simulink model "LUGOT"  (R2021a)
settings: Solver=FixedStepDiscrete  StartTime=0.0  StopTime=length(time_uwb)-1  FixedStep=Ts  MaxStep=Ts  RelTol=1e-3
values from neighbouring files (symbols this model uses):
  a = (vx .* ax + vy .* ay) ./ v    [relative_spd_vs_residual.m]    (also in smoothing_spline_fit.m)
  num_init_steps = uint8(3)    [main.m]
  outlier_threshold = standerd_deviation * 3.75 * 2 + 0.0    [main.m]
  Ts = 1.    (= 1)    [main.m]    (also in stateTransitionFcn_PF.m = 0.01)
undefined symbols (not defined in the file or in its folder): delta_h, Discrete, Time
libraries: sharedTrackingLibrary x9, simulink x6, dspstat3 x4, ctrlSharedLib x1
(part 2 of 2)

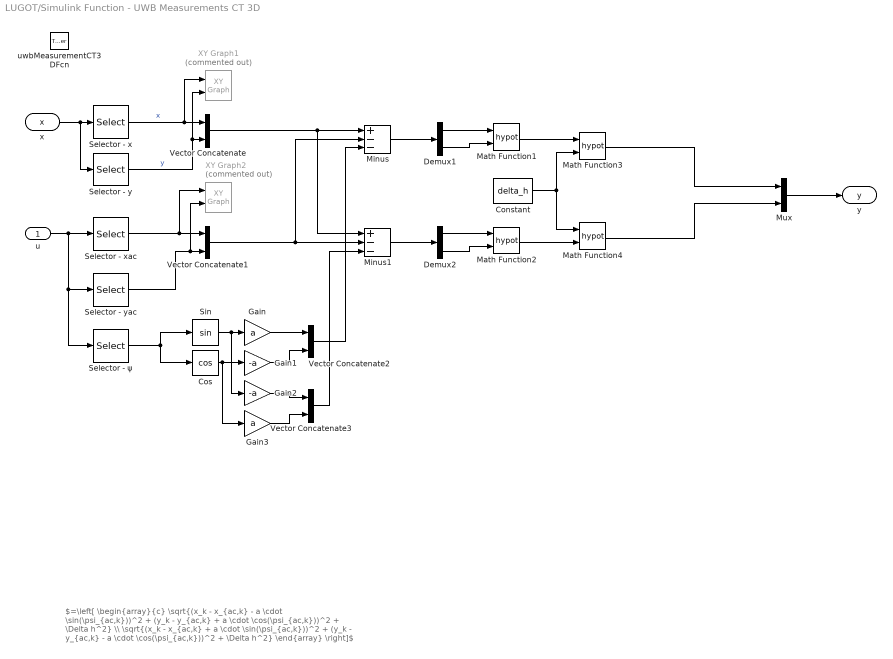
== system LUGOT/Simulink Function - UWB Measurements CT 3D ==
  note: $=\left[ \begin{array}{c} \sqrt{(x_k - x_{ac,k} - a \cdot \sin(\psi_{ac,k}))^2 + (y_k - y_{ac,k} + a \cdot \cos(\psi_{ac,k}))^2 + \Delta h^2} \\ \sqrt{(x_k - x_{ac,k} + a \cdot \sin(\psi_{ac,k}))^2 + (y_k - y_{ac,k} - a \cdot \cos(\psi_{ac,k}))^2 + \Delta h^2} \end{array} \right]$
  u : Inport
  uwbMeasurementCT3DFcn : TriggerPort  TriggerType=function-call  IsSimulinkFunction=on  FunctionName=uwbMeasurementCT3DFcn  VariantControl=Variant
  Constant : Constant  Value=delta_h
  Cos : Trigonometry  Operator=cos
  Demux1 : Demux  Outputs=2
  Demux2 : Demux  Outputs=2
  Gain : Gain  Gain=a
  Gain1 : Gain  Gain=-a
  Gain2 : Gain  Gain=-a
  Gain3 : Gain  Gain=a
  Math Function{1..4} (4 alike) : Math  Operator=hypot  SignedPower=on  SaturateOnIntegerOverflow=on
  Minus : Sum  Inputs=+--
  Minus1 : Sum  Inputs=+--
  Mux : Mux  Inputs=2
  Selector - x : Selector  InputPortWidth=5  IndexOptions=Index vector (dialog)  Indices=1  OutputSizes=1
  Selector - xac : Selector  InputPortWidth=3  IndexOptions=Index vector (dialog)  Indices=1  OutputSizes=1
  Selector - y : Selector  InputPortWidth=5  IndexOptions=Index vector (dialog)  Indices=3  OutputSizes=1
  Selector - yac : Selector  InputPortWidth=3  IndexOptions=Index vector (dialog)  Indices=2  OutputSizes=1
  Selector - ψ : Selector  InputPortWidth=3  IndexOptions=Index vector (dialog)  Indices=3  OutputSizes=1
  Sin : Trigonometry
  Vector Concatenate{,1..3} (4 alike) : Concatenate
  XY Graph1 : simulink/Sinks/XY Graph  Commented=on  xmin=0  xmax=220  ymin=-17  ymax=34  st=-1
  XY Graph2 : simulink/Sinks/XY Graph  Commented=on  xmin=0  xmax=220  ymin=-17  ymax=34  st=-1
  x : ArgIn  DisableCoverage=on  PortDimensions=5  ArgumentName=x
  y : ArgOut  DisableCoverage=on  PortDimensions=2  ArgumentName=y
  wires:
  Mux/1 -> y/1
  Minus1/1 -> Demux2/1
  Demux2/1 -> Math Function2/1
  Demux2/2 -> Math Function2/2
  Demux1/2 -> Math Function1/2
  Demux1/1 -> Math Function1/1
  Minus/1 -> Demux1/1
  Vector Concatenate3/1 -> Minus1/3
  Vector Concatenate2/1 -> Minus/3
  Vector Concatenate1/1 -> Minus1/2, Minus/2
  Vector Concatenate/1 -> Minus/1, Minus1/1
  Gain2/1 -> Vector Concatenate3/1
  Cos/1 -> Gain1/1, Gain3/1
  Sin/1 -> Gain/1, Gain2/1
  Gain3/1 -> Vector Concatenate3/2
  Gain1/1 -> Vector Concatenate2/2
  Gain/1 -> Vector Concatenate2/1
  Selector - ψ/1 -> Cos/1, Sin/1
  Selector - yac/1 -> Vector Concatenate1/2, XY Graph2/2
  Selector - xac/1 -> Vector Concatenate1/1, XY Graph2/1
  u/1 -> Selector - xac/1, Selector - yac/1, Selector - ψ/1
  x/1 -> Selector - x/1, Selector - y/1
  Selector - y/1 -> Vector Concatenate/2, XY Graph1/2  "y"
  Selector - x/1 -> Vector Concatenate/1, XY Graph1/1  "x"
  Math Function1/1 -> Math Function3/1
  Math Function2/1 -> Math Function4/2
  Constant/1 -> Math Function3/2, Math Function4/1
  Math Function3/1 -> Mux/1
  Math Function4/1 -> Mux/2

== system LUGOT/Subsystem ==
  Ts : Inport
  Constant1 : Constant  Value=[1 0 0 0; 0 1 0 0]  VectorParams1D=off
  MATLAB Function : MATLAB Function  TreatAsAtomicUnit=on
  MATLAB Function1 : MATLAB Function  TreatAsAtomicUnit=on
  A : Outport
  C : Outport  Port=2
  G : Outport  Port=3
  wires:
  MATLAB Function1/1(G) -> G/1
  Ts/1 -> MATLAB Function1/1(Ts), MATLAB Function/1(Ts)
  MATLAB Function/1(A) -> A/1
  Constant1/1 -> C/1

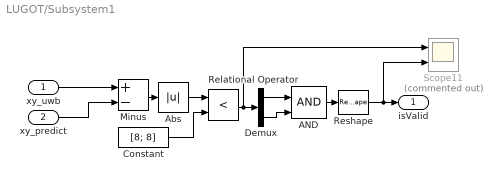
== system LUGOT/Subsystem1 ==
  xy_uwb : Inport
  xy_predict : Inport  Port=2
  AND : Logic  IconShape=distinctive  AllPortsSameDT=off  OutDataTypeStr=boolean
  Abs : Abs
  Constant : Constant  Value=[8; 8]
  Demux : Demux  Outputs=2
  Minus : Sum  Inputs=+-
  Relational Operator : RelationalOperator  Operator=<  OutDataTypeStr=boolean  RndMeth=Simplest
  Reshape : Reshape
  Scope11 : Scope  Commented=on  NumInputPorts=2
  isValid : Outport
  wires:
  Abs/1 -> Relational Operator/1
  AND/1 -> Reshape/1
  Demux/2 -> AND/2
  Constant/1 -> Relational Operator/2
  Relational Operator/1 -> Scope11/1, Demux/1
  Demux/1 -> AND/1
  xy_uwb/1 -> Minus/1
  Minus/1 -> Abs/1
  xy_predict/1 -> Minus/2
  Reshape/1 -> Scope11/2, isValid/1

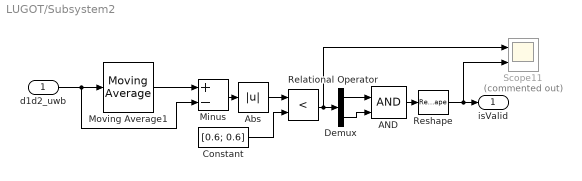
== system LUGOT/Subsystem2 ==
  d1d2_uwb : Inport
  AND : Logic  IconShape=distinctive  AllPortsSameDT=off  OutDataTypeStr=boolean
  Abs : Abs
  Constant : Constant  Value=[0.6; 0.6]
  Demux : Demux  Outputs=2
  Minus : Sum  Inputs=+-
  Moving Average1 : dspstat3/Moving Average  Method=Sliding window  ForgettingFactorPort=off  SpecifyWindowLength=on  WindowLength=20  ForgettingFactor=0.9  SimulateUsing=Code generation
  Relational Operator : RelationalOperator  Operator=<  OutDataTypeStr=boolean  RndMeth=Simplest
  Reshape : Reshape
  Scope11 : Scope  Commented=on  NumInputPorts=2
  isValid : Outport
  wires:
  Reshape/1 -> isValid/1, Scope11/2
  Minus/1 -> Abs/1
  Moving Average1/1 -> Minus/1
  Demux/1 -> AND/1
  Relational Operator/1 -> Demux/1, Scope11/1
  Constant/1 -> Relational Operator/2
  Demux/2 -> AND/2
  AND/1 -> Reshape/1
  Abs/1 -> Relational Operator/1
  d1d2_uwb/1 -> Minus/2, Moving Average1/1

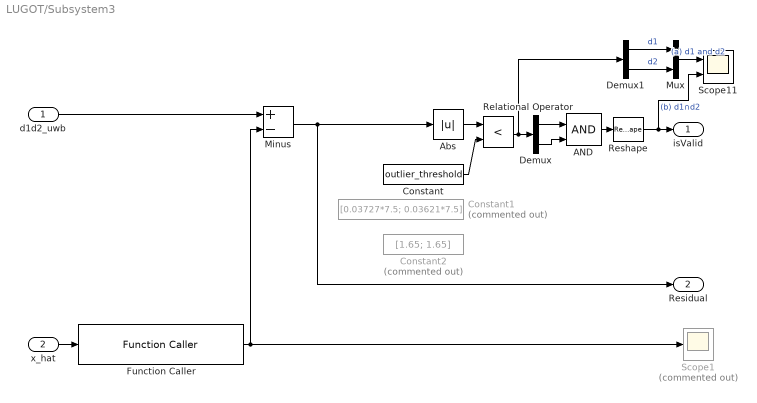
== system LUGOT/Subsystem3 ==
  d1d2_uwb : Inport
  x_hat : Inport  Port=2
  AND : Logic  IconShape=distinctive  AllPortsSameDT=off  OutDataTypeStr=boolean
  Abs : Abs
  Constant : Constant  Value=outlier_threshold
  Constant1 : Constant  Commented=on  Value=[0.03727*7.5; 0.03621*7.5]
  Constant2 : Constant  Commented=on  Value=[1.65; 1.65]
  Demux : Demux  Outputs=2
  Demux1 : Demux  Outputs=2
  Function Caller : FunctionCaller  FunctionPrototype=y = uwbMeasurementCT3DFcn(x)  InputArgumentSpecifications=<Enter example>  OutputArgumentSpecifications=<Enter example>
  Minus : Sum  Inputs=+-
  Mux : Mux  Inputs=2
  Relational Operator : RelationalOperator  Operator=<  OutDataTypeStr=boolean  RndMeth=Simplest
  Reshape : Reshape
  Scope1 : Scope  Commented=on
  Scope11 : Scope  NumInputPorts=2
  isValid : Outport
  Residual : Outport  Port=2
  wires:
  Abs/1 -> Relational Operator/1
  AND/1 -> Reshape/1
  Demux/2 -> AND/2
  Constant/1 -> Relational Operator/2
  Relational Operator/1 -> Demux1/1, Demux/1
  Demux/1 -> AND/1
  d1d2_uwb/1 -> Minus/1
  Minus/1 -> Abs/1, Residual/1
  Reshape/1 -> Scope11/2, isValid/1  "(b) d1∩d2"
  Function Caller/1 -> Scope1/1, Minus/2
  x_hat/1 -> Function Caller/1
  Mux/1 -> Scope11/1  "(a) d1 and d2"
  Demux1/1 -> Mux/1  "d1"
  Demux1/2 -> Mux/2  "d2"

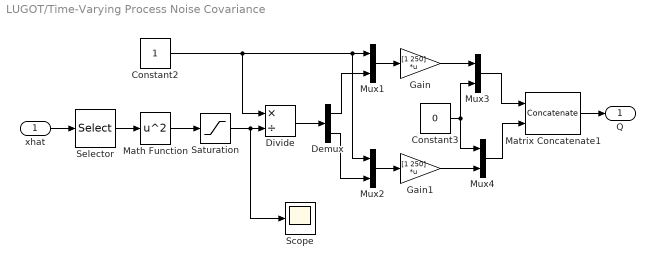
== system LUGOT/Time-Varying Process Noise Covariance ==
  xhat : Inport
  Constant2 : Constant
  Constant3 : Constant  Value=0
  Demux : Demux  Outputs=2
  Divide : Product  Inputs=*/
  Gain : Gain  Gain=[1 250]  Multiplication=Matrix(K*u)
  Gain1 : Gain  Gain=[1 250]  Multiplication=Matrix(K*u)
  Math Function : Math  Operator=square  SignedPower=on  SaturateOnIntegerOverflow=on
  Matrix Concatenate1 : Concatenate  Mode=Multidimensional array  ConcatenateDimension=2
  Mux{1..4} (4 alike) : Mux  Inputs=2
  Saturation : Saturate  UpperLimit=625  LowerLimit=25
  Scope : Scope
  Selector : Selector  InputPortWidth=4  IndexOptions=Index vector (dialog)  Indices=[3 4]  OutputSizes=1
  Q : Outport
  wires:
  Selector/1 -> Math Function/1
  xhat/1 -> Selector/1
  Saturation/1 -> Scope/1, Divide/2
  Constant2/1 -> Mux2/1, Mux1/1, Divide/1
  Divide/1 -> Demux/1
  Gain/1 -> Mux3/1
  Constant3/1 -> Mux3/2, Mux4/1
  Mux3/1 -> Matrix Concatenate1/1
  Mux4/1 -> Matrix Concatenate1/2
  Matrix Concatenate1/1 -> Q/1
  Demux/1 -> Mux1/2
  Demux/2 -> Mux2/2
  Mux1/1 -> Gain/1
  Mux2/1 -> Gain1/1
  Gain1/1 -> Mux4/2
  Math Function/1 -> Saturation/1

== system LUGOT/calc ΔT ==
  Time : Inport
  Enable : EnablePort
  Constant1 : Constant  Commented=on  Value=1/120
  Memory : Memory  InitialCondition=-1/120  InheritSampleTime=on
  Subtract : Sum  Inputs=+-
  Switch : Switch  Commented=on  Criteria=u2 > Threshold  Threshold=1e-3
  dt : Outport
  wires:
  Subtract/1 -> dt/1
  Time/1 -> Memory/1, Subtract/1
  Memory/1 -> Subtract/2
  ? -> Switch/1, Switch/2
  Constant1/1 -> Switch/3

== system LUGOT/calc ΔT1 ==
  Time : Inport
  Enable : EnablePort
  Memory : Memory  InitialCondition=-1/120  InheritSampleTime=on
  Subtract : Sum  Inputs=+-
  dt : Outport
  wires:
  Subtract/1 -> dt/1
  Time/1 -> Memory/1, Subtract/1
  Memory/1 -> Subtract/2

== system LUGOT/initial_counter ==
  Enable : EnablePort
  Add : Sum
  Constant : Constant
  Constant2 : Constant  Value=num_init_steps
  Memory2 : Memory  InheritSampleTime=on
  Relational Operator : RelationalOperator  Operator=>  OutDataTypeStr=boolean  RndMeth=Simplest
  Scope27 : Scope  Commented=on
  Out1 : Outport
  wires:
  Constant2/1 -> Relational Operator/2
  Constant/1 -> Add/1
  Add/1 -> Memory2/1, Scope27/1, Relational Operator/1
  Memory2/1 -> Add/2
  Relational Operator/1 -> Out1/1

== matlab function LUGOT/Simulink Function - State Transition CTRV/MATLAB Function ==
  data: current_state input; next_state output; dt input
% https://blog.csdn.net/west_gege/article/details/121405259
% function state  = predict_omega(state,dt)
%   % state = x,y,v,theta,omega
%   state(1) = state(1) + (state(3) / state(5)) * (sin(state(4) + state(5) * dt) - sin(state(4)));
%   state(2) = state(2) + (state(3) / state(5)) *(-cos(state(4) + state(5) * dt) + cos(state(4)));
%   state(3) = state(3);
%   state(4) = state(4) + state(5) * dt;
%   state(5) = state(5);
% end
% 
% function [state] = predict_omega(state,dt)
%     % state = x,y,v,theta,omega
%   state(1) = state(1) + state(3)*cos(state(4))*dt;
%   state(2) = state(2) + state(3)*sin(state(4))*dt;
%   state(3) = state(3);
%   state(4) = state(4);
%   state(5) = state(5);
% end

function next_state = ctrv_transition(current_state, dt)
    % 解析当前状态
    x = current_state(1);
    y = current_state(2);
    theta = current_state(3);
    v = current_state(4);
    omega = current_state(5);

    % 如果转向率非零，则使用CTRV模型进行状态更新
    if omega ~= 0
        % 计算新的位置和航向
        next_x = x + (v/omega) * (sin(theta + omega*dt) - sin(theta));
        next_y = y + (v/omega) * (cos(theta) - cos(theta + omega*dt));
        next_theta = theta + omega*dt;
    else
        % 当转向率为零时，退化为直线运动
        next_x = x + v*cos(theta)*dt;
        next_y = y + v*sin(theta)*dt;
        next_theta = theta;
    end

    % 更新速度和转向率（这里假设它们在时间间隔内保持不变）
    next_v = v;
    next_omega = omega;

    % 组合成新的状态向量
    next_state = [next_x; next_y; next_theta; next_v; next_omega];
end

== matlab function LUGOT/Simulink Function - State Transition CT/MATLAB Function ==
  data: x input; y output; w input; dt input
function y = stateTransitionCTFcn(x,w,dt)

y = constturn(x,w,dt); %0.01

== matlab function LUGOT/Simulink Function - State Transition Jacobian CT/MATLAB Function ==
  data: x input; A output; w input; G output; dt input
function [A,G] = fcn(x,w,dt)
[A,G] = constturnjac(x,w,dt); % 0.01

== matlab function LUGOT/Simulink Function - UWB Measurement Jacobian CT/MATLAB Function ==
  data: X input; H output; x_ac input; y_ac input; psi_ac input; a input
% function C = uwbMeasurementJacobianCTFcn(x, xac, yac, psi_ac, a)
%     % 输入参数：
%     % x : 状态向量 [px; py; v; psi; psidot]
%     % xac, yac : 自车的坐标
%     % psi_ac : 自车的朝向
%     % a : 基站距离的一半，单位m
% 
%     % 提取状态变量
%     px = x(1);
%     py = x(2);
% 
%     % 小正数epsilon，防止除零错误
%     epsilon = 1e-6;
% 
%     % 计算观测函数的两部分距离
%     r1 = sqrt((px - xac - a * sin(psi_ac))^2 + (py - yac + a * cos(psi_ac))^2);
%     r2 = sqrt((px - xac + a * sin(psi_ac))^2 + (py - yac - a * cos(psi_ac))^2);
% 
%     % 防止r1或r2为零的情况
%     r1 = max(r1, epsilon);
%     r2 = max(r2, epsilon);
% 
%     % 雅可比矩阵的第一行
%     Hk11 = (px - xac - a * sin(psi_ac)) / r1;
%     Hk12 = (py - yac + a * cos(psi_ac)) / r1;
% 
%     % 雅可比矩阵的第二行
%     Hk21 = (px - xac + a * sin(psi_ac)) / r2;
%     Hk22 = (py - yac - a * cos(psi_ac)) / r2;
% 
%     % 组装完整的雅可比矩阵
%     Hk = [Hk11, Hk12, 0, 0, 0;
%           Hk21, Hk22, 0, 0, 0];
%     C = Hk;
% end

%%%%%%%%%%%%%%%%%%%%%%%%%%%%%%%%%%%%%%%%%%%%%%%%%%%%%%%%%%%%%%%%%%%%%%%%%%%%%%%%%%%%%%%%%%%
% function H = calculateJacobian(X, x_ac, y_ac, psi_ac, a)
%     px = X(1);
%     py = X(2);
%     
%     % 计算两个距离
%     h1 = sqrt((px - x_ac - a * sin(psi_ac))^2 + (py - y_ac + a * cos(psi_ac))^2);
%     h2 = sqrt((px - x_ac + a * sin(psi_ac))^2 + (py - y_ac - a * cos(psi_ac))^2);
%     
%     % 计算雅可比矩阵的各个元素
%     H = zeros(2, 5);
%     H(1, 1) = (px - x_ac - a * sin(psi_ac)) / h1;
%     H(1, 2) = (py - y_ac + a * cos(psi_ac)) / h1;
%     H(2, 1) = (px - x_ac + a * sin(psi_ac)) / h2;
%     H(2, 2) = (py - y_ac - a * cos(psi_ac)) / h2;
%     
%     % 其他项为0
% end
%%%%%%%%%%%%%%%%%%%%%%%%%%%%%%%%%%%%%%%%%%%%%%%%%%%%%%%%%%%%%%%%%%%%%%%%%%%%%%%%%%%%%%%%%%%%%%%%%
% function H = calculateJacobian(X, x_ac, y_ac, psi_ac, a)
%     px = X(1);
%     py = X(2);
%     epsilon = 1e-4;  % 防止除以非常小的数
% 
%     % 计算两个距离
%     r1_squared = (px - x_ac - a * sin(psi_ac))^2 + (py - y_ac + a * cos(psi_ac))^2;
%     r2_squared = (px - x_ac + a * sin(psi_ac))^2 + (py - y_ac - a * cos(psi_ac))^2;
%     h1 = sqrt(r1_squared);
%     h2 = sqrt(r2_squared);
% 
%     % 计算雅可比矩阵的各个元素
%     H = zeros(2, 5);
%     if r1_squared >= epsilon^2
%         H(1, 1) = (px - x_ac - a * sin(psi_ac)) / h1;
%         H(1, 2) = (py - y_ac + a * cos(psi_ac)) / h1;
%     end
%     if r2_squared >= epsilon^2
%         H(2, 1) = (px - x_ac + a * sin(psi_ac)) / h2;
%         H(2, 2) = (py - y_ac - a * cos(psi_ac)) / h2;
%     end
% 
%     % 如果 r1 或 r2 接近零，则对应的雅可比矩阵行设置为零
%     if r1_squared < epsilon^2
%         H(1, :) = 0;
%     end
%     if r2_squared < epsilon^2
%         H(2, :) = 0;
%     end
% end
%%%%%%%%%%%%%%%%%%%%%%%%%%%%%%%%%%%%%%%%%%%%%%%%%%%%%%%%%%%%%%%%%%%%%%%%%%%%%%%%%%%%%%%%%%
function H = calculateJacobian(X, x_ac, y_ac, psi_ac, a)
    px = X(1);
    py = X(2);
    epsilon = 1e-4;  % 防止除以接近零的数

    % 计算两个距离
    r1_squared = (px - x_ac - a * sin(psi_ac))^2 + (py - y_ac + a * cos(psi_ac))^2;
    r2_squared = (px - x_ac + a * sin(psi_ac))^2 + (py - y_ac - a * cos(psi_ac))^2;

    % 防止除零
    r1_squared = max(r1_squared, epsilon^2);
    r2_squared = max(r2_squared, epsilon^2);

    h1 = sqrt(r1_squared);
    h2 = sqrt(r2_squared);

    % 计算雅可比矩阵的各个元素
    H = zeros(2, 5);
    H(1, 1) = (px - x_ac - a * sin(psi_ac)) / h1;
    H(1, 2) = (py - y_ac + a * cos(psi_ac)) / h1;
    H(2, 1) = (px - x_ac + a * sin(psi_ac)) / h2;
    H(2, 2) = (py - y_ac - a * cos(psi_ac)) / h2;

    % 状态向量中的速度v，角度ψ和角速度ψ̇的偏导数是0，因为它们不影响测量的距离
end

== matlab function LUGOT/Simulink Function - UWB Measurement Jacobian CT 3D/MATLAB Function ==
  data: X input; H output; x_ac input; y_ac input; psi_ac input; a input; delta_h input
function H = calculateJacobian(X, x_ac, y_ac, psi_ac, a, delta_h)
    px = X(1);
    py = X(2);
    epsilon = 1e-4;  % 防止除以接近零的数

    % 计算两个距离
    r1_squared = (px - x_ac - a * sin(psi_ac))^2 + (py - y_ac + a * cos(psi_ac))^2 + delta_h^2;
    r2_squared = (px - x_ac + a * sin(psi_ac))^2 + (py - y_ac - a * cos(psi_ac))^2 + delta_h^2;

    % 防止除零
    r1_squared = max(r1_squared, epsilon^2);
    r2_squared = max(r2_squared, epsilon^2);

    h1 = sqrt(r1_squared);
    h2 = sqrt(r2_squared);

    % 计算雅可比矩阵的各个元素
    H = zeros(2, 5);
    H(1, 1) = (px - x_ac - a * sin(psi_ac)) / h1;
    H(1, 2) = (py - y_ac + a * cos(psi_ac)) / h1;
    H(2, 1) = (px - x_ac + a * sin(psi_ac)) / h2;
    H(2, 2) = (py - y_ac - a * cos(psi_ac)) / h2;

    % 状态向量中的速度v，角度ψ和角速度ψ̇的偏导数是0，因为它们不影响测量的距离
end

== matlab function LUGOT/Subsystem/MATLAB Function ==
  data: Ts input; A output
function A = f(Ts)
    A = [1 0 Ts 0; 0 1 0 Ts; 0 0 1 0; 0 0 0 1];
end

== matlab function LUGOT/Subsystem/MATLAB Function1 ==
  data: Ts input; G output
function G = f(Ts)
    G = [Ts/2 0; 0 Ts/2; 1 0; 0 1];
end

== matlab function LUGOT/Simulink Function - State Transition CT1/MATLAB Function ==
  data: x input; y output; w input; dt input
function y = stateTransitionCTFcn(x,w,dt)

y = constturn(x,w,dt); %0.01

== matlab function LUGOT/Simulink Function - State Transition Jacobian CT1/MATLAB Function ==
  data: x input; A output; w input; G output; dt input
function [A,G] = fcn(x,w,dt)
[A,G] = constturnjac(x,w,dt); % 0.01

== matlab function LUGOT/MATLAB Function ==
  data: x input; D output; mu input; Sigma input
function D = mahalanobisDistance(x, mu, Sigma)
    % 计算马氏距离
    % x - 数据点
    % mu - 均值向量
    % Sigma - 协方差矩阵

    if det(Sigma) == 0
        error('协方差矩阵Sigma不能是奇异的');
    end

    Sigma_inv = inv(Sigma); % 计算协方差矩阵的逆
    diff = x - mu;
    D = sqrt(diff' * Sigma_inv * diff);
end
